simulink model "actuators_monitor_func"  (R2021a)
settings: Solver=VariableStepAuto  StartTime=0.0  StopTime=10.0  RelTol=1e-3
settings Model: Creator=Intuito_PC  LastModifiedBy=Intuito_PC

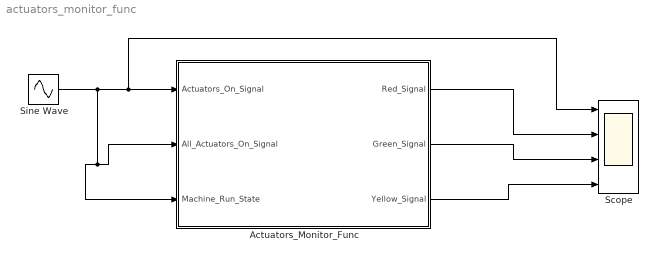
== system actuators_monitor_func ==
  Actuators_Monitor_Func : MATLAB Function  TreatAsAtomicUnit=on
  Scope : Scope  NumInputPorts=4
  Sine Wave : Sin  SampleTime=0
  wires:
  Sine Wave/1 -> Actuators_Monitor_Func/3(Machine_Run_State), Actuators_Monitor_Func/2(All_Actuators_On_Signal), Scope/1, Actuators_Monitor_Func/1(Actuators_On_Signal)
  Actuators_Monitor_Func/3(Yellow_Signal) -> Scope/4
  Actuators_Monitor_Func/2(Green_Signal) -> Scope/3
  Actuators_Monitor_Func/1(Red_Signal) -> Scope/2

== matlab function actuators_monitor_func/Actuators_Monitor_Func ==
  data: Actuators_On_Signal input; Red_Signal output; All_Actuators_On_Signal input; Machine_Run_State input; Green_Signal output; Yellow_Signal output
function [Red_Signal, Green_Signal, Yellow_Signal] = fcn(Actuators_On_Signal, All_Actuators_On_Signal, Machine_Run_State)
if Actuators_On_Signal > 0
%     Light yellow
        Yellow_Signal = 1;
else
    %     Light yellow off
        Yellow_Signal = 0;
end
if All_Actuators_On_Signal > 0
%     Light Red
        Red_Signal = 1;
else
    %     Light Red off
        Red_Signal = 0;
end
if Machine_Run_State == 0
%     Light Green in standby
        Green_Signal = 1;
else
    %     Light yellow oof
        Green_Signal = 0;
end
end
